simulink model "nav_leha19b"  (R2019b)
settings: Solver=FixedStepDiscrete  StartTime=0.0  StopTime=2500  FixedStep=dT  RelTol=1e-3
values from neighbouring files (symbols this model uses):
  al_gp_M = k    (= 2)    [gnss_data_orig.m]
  al_gp_max = 15    [model_nav_system_flight_simulation_orig.m]
  al_gp_mu = 3.986004418E+14    (= 398600441800000)    [gnss_data_orig.m]
  al_gp_resolution = 1000    [gnss_data_orig.m]
  al_gp_t0 = gnss_strings_2(1,4)    [gnss_data_orig.m]
  dT = 1    [model_nav_system_flight_simulation_orig.m]
  mean_p_ion = 1.3    [model_nav_system_flight_simulation_orig.m]
  mean_p_trop = 0.3    [model_nav_system_flight_simulation_orig.m]
  P0_b_g = zeros(23,23)    [model_nav_system_flight_simulation_orig.m]
  P_b = zeros(21, 21)    [model_nav_system_flight_simulation_orig.m]
  R_a = 6378136    [model_nav_system_flight_simulation_orig.m]
  R_betta = 0.0053171    [model_nav_system_flight_simulation_orig.m]
  R_betta1 = 71 * 10^-7    (= 7.1e-06)    [model_nav_system_flight_simulation_orig.m]
  R_e2 = 0    [model_nav_system_flight_simulation_orig.m]
  R_ge = 9.78049    [model_nav_system_flight_simulation_orig.m]
  R_q = 0.00346775    [model_nav_system_flight_simulation_orig.m]
  R_u = 7.292115*10^(-5)    (= 7.292115e-05)    [model_nav_system_flight_simulation_orig.m]
  sigma_error_acs0 = [SKO_del_n_x SKO_del_n_y SKO_del_n_z]    [model_nav_system_flight_simulation_orig.m]
  sigma_error_DUS0 = [SKO_del_Omega_x SKO_del_Omega_y SKO_del_Omega_z]    [model_nav_system_flight_simulation_orig.m]
  sigma_gnss0 = SKO_p_del_T + SKO_p_del_t + mean_p_ion + mean_p_trop + SKO_p_mnogoluch + SKO_p_noise    (= 5.61)    [model_nav_system_flight_simulation_orig.m]
  SKO_p_del_T = 3    [model_nav_system_flight_simulation_orig.m]
  SKO_p_del_t = 0.01    [model_nav_system_flight_simulation_orig.m]
  SKO_p_mnogoluch = 0.5    [model_nav_system_flight_simulation_orig.m]
  SKO_p_noise = 0.5    [model_nav_system_flight_simulation_orig.m]
  tr_H = flight_mission(3,1)    [model_nav_system_flight_simulation_orig.m]
  W = W'    [model_nav_system_flight_simulation_orig.m]
  X0 = X0'    [model_nav_system_flight_simulation_orig.m]
  X0_b_g = X0_b_g * 0    [model_nav_system_flight_simulation_orig.m]
undefined symbols (not defined in the file or in its folder): al_gp_e, al_gp_health, al_gp_i, al_gp_lan, al_gp_m0, al_gp_sqrt_a, al_gp_w, sigma_error_D_p, sigma_error_D_p1, sigma_gnss0_0, tr_course, tr_fi, tr_la, tr_pitch, tr_roll, tr_V_E, tr_V_H, tr_V_N, tr_X_dgsk, tr_Y_dgsk, tr_Z_dgsk
libraries: simulink_extras x8
(part 2 of 3)

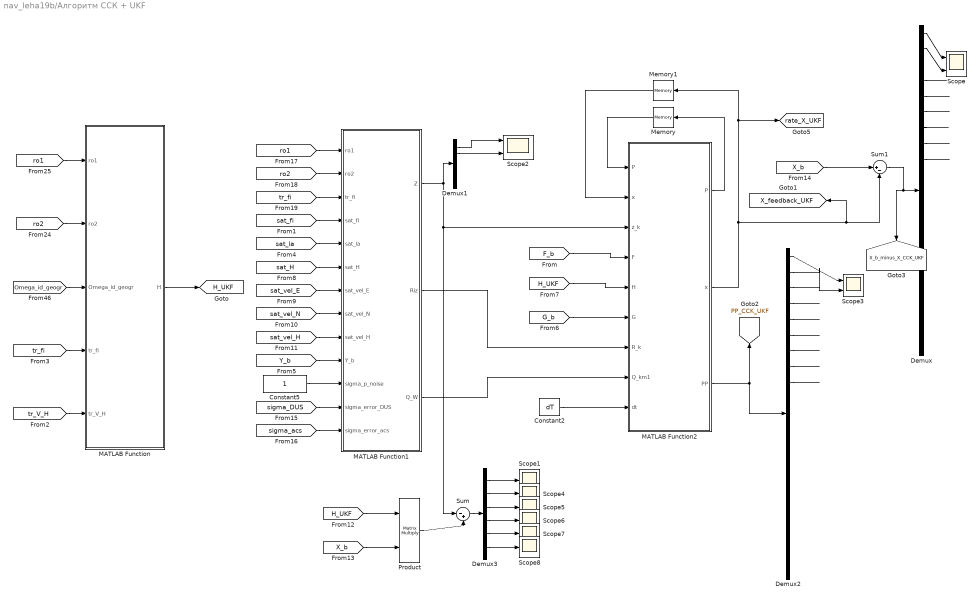
== system nav_leha19b/Алгоритм ССК + UKF ==
  Constant2 : Constant  Value=dT
  Constant5 : Constant
  Demux : Demux  Outputs=21
  Demux1 : Demux  Outputs=6
  Demux2 : Demux  Outputs=21
  Demux3 : Demux  Outputs=6
  MATLAB Function : MATLAB Function  TreatAsAtomicUnit=on
  MATLAB Function1 : MATLAB Function  TreatAsAtomicUnit=on
  MATLAB Function2 : MATLAB Function  TreatAsAtomicUnit=on
  Memory : Memory  InitialCondition=P_b
  Memory1 : Memory  InitialCondition=X0
  Product : Product  Multiplication=Matrix(*)
  Scope : Scope  NumInputPorts=2
  Scope{1,4..8} (6 alike) : Scope
  Scope2 : Scope  NumInputPorts=2
  Scope3 : Scope  NumInputPorts=2
  Sum : Sum  Inputs=|-+
  Sum1 : Sum  Inputs=|+-
  tag scope: H_UKF=global, PP_CCK_UKF=global, X_b_minus_X_CCK_UKF=global, X_feedback_UKF=global, rate_X_UKF=global
  wires:
  Constant2/1 -> MATLAB Function2/9(dt)
  [G_b] -> MATLAB Function2/6(G)
  [H_UKF] -> MATLAB Function2/5(H)
  MATLAB Function/1(H) -> [H_UKF]
  [ro2] -> MATLAB Function/2(ro2)
  [ro1] -> MATLAB Function/1(ro1)
  [Omega_id_geogr] -> MATLAB Function/3(Omega_id_geogr)
  [tr_fi] -> MATLAB Function/4(tr_fi)
  [tr_V_H] -> MATLAB Function/5(tr_V_H)
  [Y_b] -> MATLAB Function1/10(Y_b)
  [sigma_DUS] -> MATLAB Function1/12(sigma_error_DUS)
  [sigma_acs] -> MATLAB Function1/13(sigma_error_acs)
  MATLAB Function1/1(Z) -> Demux1/1, Sum/1, MATLAB Function2/3(z_k)
  MATLAB Function1/2(Riz) -> MATLAB Function2/7(R_k)
  MATLAB Function1/3(Q_W) -> MATLAB Function2/8(Q_km1)
  [X_b] -> Sum1/1
  Sum1/1 -> Demux/1, [X_b_minus_X_CCK_UKF]
  [sat_fi] -> MATLAB Function1/4(sat_fi)
  [sat_la] -> MATLAB Function1/5(sat_la)
  [sat_H] -> MATLAB Function1/6(sat_H)
  [sat_vel_N] -> MATLAB Function1/8(sat_vel_N)
  [sat_vel_H] -> MATLAB Function1/9(sat_vel_H)
  [sat_vel_E] -> MATLAB Function1/7(sat_vel_E)
  Constant5/1 -> MATLAB Function1/11(sigma_p_noise)
  Demux1/1 -> Scope2/1
  Demux1/2 -> Scope2/2
  Demux/4 -> ?
  Demux/5 -> ?
  Demux/6 -> ?
  Demux/7 -> ?
  Demux/8 -> ?
  Demux/9 -> ?
  Demux2/1 -> Scope3/1
  Demux2/2 -> Scope3/2
  Demux2/3 -> ?
  Demux2/4 -> ?
  Demux2/5 -> ?
  Demux2/6 -> ?
  Demux2/7 -> ?
  Demux2/8 -> ?
  Demux2/9 -> ?
  Demux/1 -> Scope/1
  Demux/2 -> Scope/2
  Product/1 -> Sum/2
  [H_UKF] -> Product/1
  [X_b] -> Product/2
  Sum/1 -> Demux3/1
  Demux3/1 -> Scope1/1
  Demux3/2 -> Scope4/1
  Demux3/3 -> Scope5/1
  Demux3/4 -> Scope6/1
  Demux3/5 -> Scope7/1
  Demux3/6 -> Scope8/1
  [ro1] -> MATLAB Function1/1(ro1)
  [ro2] -> MATLAB Function1/2(ro2)
  [F_b] -> MATLAB Function2/4(F)
  MATLAB Function2/1(P) -> Memory/1
  Memory/1 -> MATLAB Function2/1("P ")
  MATLAB Function2/2(x) -> [X_feedback_UKF], Sum1/2, Memory1/1, [rate_X_UKF]
  Memory1/1 -> MATLAB Function2/2("x ")
  MATLAB Function2/3(PP) -> Demux2/1, [PP_CCK_UKF]
  [tr_fi] -> MATLAB Function1/3(tr_fi)

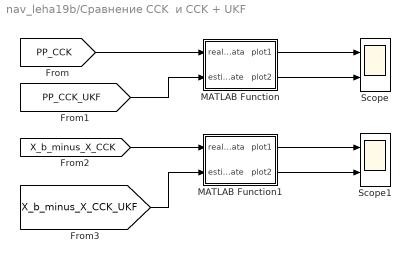
== system nav_leha19b/Сравнение ССK  и CCK + UKF ==
  MATLAB Function : MATLAB Function  TreatAsAtomicUnit=on
  MATLAB Function1 : MATLAB Function  TreatAsAtomicUnit=on
  Scope : Scope  NumInputPorts=2
  Scope1 : Scope  NumInputPorts=2
  wires:
  [PP_CCK] -> MATLAB Function/1(real_data)
  MATLAB Function/1(plot1) -> Scope/1
  [X_b_minus_X_CCK_UKF] -> MATLAB Function1/2(estimate)
  [PP_CCK_UKF] -> MATLAB Function/2(estimate)
  [X_b_minus_X_CCK] -> MATLAB Function1/1(real_data)
  MATLAB Function/2(plot2) -> Scope/2
  MATLAB Function1/1(plot1) -> Scope1/1
  MATLAB Function1/2(plot2) -> Scope1/2

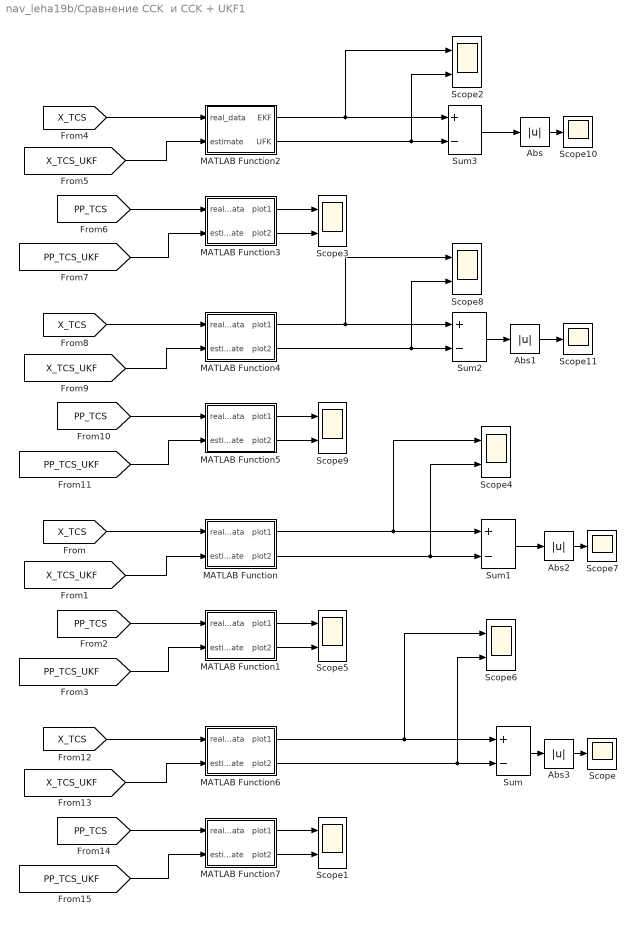
== system nav_leha19b/Сравнение ССK  и CCK + UKF1 ==
  Abs{,1..3} (4 alike) : Abs
  MATLAB Function : MATLAB Function  TreatAsAtomicUnit=on
  MATLAB Function1 : MATLAB Function  TreatAsAtomicUnit=on
  MATLAB Function2 : MATLAB Function  TreatAsAtomicUnit=on
  MATLAB Function3 : MATLAB Function  TreatAsAtomicUnit=on
  MATLAB Function4 : MATLAB Function  TreatAsAtomicUnit=on
  MATLAB Function5 : MATLAB Function  TreatAsAtomicUnit=on
  MATLAB Function6 : MATLAB Function  TreatAsAtomicUnit=on
  MATLAB Function7 : MATLAB Function  TreatAsAtomicUnit=on
  Scope{,7,10..11} (4 alike) : Scope
  Scope{1..6,8..9} (8 alike) : Scope  NumInputPorts=2
  Sum{,1..3} (4 alike) : Sum  Inputs=+-
  wires:
  [PP_TCS] -> MATLAB Function1/1(real_data)
  MATLAB Function1/1(plot1) -> Scope5/1
  MATLAB Function1/2(plot2) -> Scope5/2
  [PP_TCS_UKF] -> MATLAB Function1/2(estimate)
  [X_TCS] -> MATLAB Function/1(real_data)
  [X_TCS_UKF] -> MATLAB Function/2(estimate)
  [X_TCS_UKF] -> MATLAB Function2/2(estimate)
  [PP_TCS_UKF] -> MATLAB Function3/2(estimate)
  [X_TCS] -> MATLAB Function2/1(real_data)
  [PP_TCS] -> MATLAB Function3/1(real_data)
  [X_TCS_UKF] -> MATLAB Function4/2(estimate)
  [PP_TCS_UKF] -> MATLAB Function5/2(estimate)
  [X_TCS] -> MATLAB Function4/1(real_data)
  MATLAB Function5/2(plot2) -> Scope9/2
  MATLAB Function5/1(plot1) -> Scope9/1
  [PP_TCS] -> MATLAB Function5/1(real_data)
  MATLAB Function6/2(plot2) -> Scope6/2, Sum/2
  [X_TCS_UKF] -> MATLAB Function6/2(estimate)
  [PP_TCS_UKF] -> MATLAB Function7/2(estimate)
  [X_TCS] -> MATLAB Function6/1(real_data)
  MATLAB Function6/1(plot1) -> Sum/1, Scope6/1
  [PP_TCS] -> MATLAB Function7/1(real_data)
  MATLAB Function/2(plot2) -> Sum1/2, Scope4/2
  MATLAB Function/1(plot1) -> Sum1/1, Scope4/1
  MATLAB Function4/2(plot2) -> Sum2/2, Scope8/2
  MATLAB Function4/1(plot1) -> Scope8/1, Sum2/1
  MATLAB Function2/2(UFK) -> Sum3/2, Scope2/2
  MATLAB Function2/1(EKF) -> Sum3/1, Scope2/1
  Sum3/1 -> Abs/1
  Abs/1 -> Scope10/1
  Sum2/1 -> Abs1/1
  Abs1/1 -> Scope11/1
  Sum1/1 -> Abs2/1
  Abs2/1 -> Scope7/1
  Abs3/1 -> Scope/1
  Sum/1 -> Abs3/1
  MATLAB Function7/2(plot2) -> Scope1/2
  MATLAB Function7/1(plot1) -> Scope1/1
  MATLAB Function3/2(plot2) -> Scope3/2
  MATLAB Function3/1(plot1) -> Scope3/1

== matlab function nav_leha19b/trajectory/MATLAB Function1 ==
  data: tr_dV_E input; tr_V_E input; tr_dV_N input; tr_V_N input; n_E output; n_N output; tr_dV_H input; n_H output; Omega_E output; Omega_N output; tr_V_H input; tr_fi input; tr_H input; R_ge input; R_betta input; R_betta1 input; R_e2 input; R_a input; R_q input; R_u input; Omega_H output; Omega1_E1 output; Omega1_N1 output; Omega1_H1 output; ro1 output; ro2 output
function [n_E, n_N, n_H, Omega_E, Omega_N, Omega_H, Omega1_E1, Omega1_N1, Omega1_H1, ro1, ro2]  = n(tr_dV_E, tr_V_E, tr_dV_N, tr_V_N, tr_dV_H, tr_V_H, tr_fi, tr_H, R_ge, R_betta, R_betta1, R_e2, R_a, R_q, R_u)

g0 = R_ge*(1 + R_betta*sin(tr_fi).^2 + R_betta1*sin(2*tr_fi).^2);
gy = g0*sin(2*tr_fi)*tr_H*(R_e2/R_a - 2*R_q)/R_a;
gz = g0 + tr_H*(3*tr_H/R_a - 2*R_q*R_ge*cos(tr_fi).^2 + R_e2*(3*sin(tr_fi).^2 - 1) - R_q*(1 + 6*sin(tr_fi).^2))/R_a;

ro1 = (R_a*(1 - R_e2)./(sqrt((1 - R_e2*sin(tr_fi).^2).^3))) + tr_H;
ro2 = (R_a./(sqrt(1 - R_e2*sin(tr_fi).^2))) + tr_H;

Omega1_E = -tr_V_N/ro1;
Omega1_N = tr_V_E/ro2;
Omega1_H = (tr_V_E/ro2)*tan(tr_fi);

u_N = R_u*cos(tr_fi);
u_H = R_u*sin(tr_fi);
Omega_E = Omega1_E;
Omega_N = Omega1_N + u_N;
Omega_H = Omega1_H + u_H;

n_E = tr_dV_E - (Omega1_H + 2*u_H)*tr_V_N + (Omega1_N + 2*u_N)*tr_V_H;
n_N = tr_dV_N + (Omega1_H + 2*u_H)*tr_V_E - Omega1_E*tr_V_H - gy;
n_H = tr_dV_H - (Omega1_N + 2*u_N)*tr_V_E + Omega1_E*tr_V_N - gz;

Omega1_E1 = -(tr_dV_N - tr_V_H*tr_V_N/ro1)/ro1;
Omega1_N1 = (tr_dV_E - R_u*sin(tr_fi)*tr_V_N - tr_V_H*tr_V_E/ro2)/ro2;
Omega1_H1 = (R_u*cos(tr_fi)*tr_V_N + n_E*tan(tr_fi) + tr_V_H*Omega_H +(tr_V_E*tr_V_N)/(ro2*cos(tr_fi).^2))/ro2;
end

== matlab function nav_leha19b/Алгоритм ССК + UKF/MATLAB Function ==
  settings: updateMethod=DISCRETE  sampleTime=dT
  data: ro1 input; H output; ro2 input; Omega_id_geogr input; tr_fi input; tr_V_H input
function H = H_b_gp(ro1, ro2,  Omega_id_geogr,  tr_fi,  tr_V_H)

    H = zeros(6,21);

    H(1,1) = 1 / (ro2 * cos(tr_fi));
    H(2,2) = 1/ro1;
    H(4,1) = - ((tr_V_H/ro2) + Omega_id_geogr(1) * tan(tr_fi));
    H(4,2) = -Omega_id_geogr(3);
    H(4,4) = 1;
    H(5,1) = - tr_V_H/ro1;
    H(5,5) = 1;

end

== matlab function nav_leha19b/trajectory/MATLAB Function2 ==
  data: tr_X_dgsk input; tr_Y_dgsk input; tr_Z_dgsk input; tr_X_dgsk1 output; tr_Y_dgsk1 output; tr_Z_dgsk1 output
function [tr_X_dgsk1, tr_Y_dgsk1, tr_Z_dgsk1] = fcn(tr_X_dgsk, tr_Y_dgsk, tr_Z_dgsk)
persistent i
if isempty (i)
    i = 1;
end
tr_X_dgsk1 = tr_X_dgsk(i);
tr_Y_dgsk1 = tr_Y_dgsk(i);
tr_Z_dgsk1 = tr_Z_dgsk(i);
i = i + 1;
end

== matlab function nav_leha19b/trajectory/MATLAB Function3 ==
  data: tr_fi input; tr_la input; tr_H input; tr_fit output; tr_lat output; tr_Ht output; tr_V_E input; tr_V_Et output; tr_V_N input; tr_V_H input; tr_V_Nt output; tr_V_Ht output; tr_course input; tr_roll input; tr_courset output; tr_yawt output; tr_rollt output; tr_pitch input; tr_pitcht output
function [tr_fit, tr_lat, tr_Ht, tr_V_Et, tr_V_Nt, tr_V_Ht, tr_courset, tr_yawt, tr_rollt, tr_pitcht] = fcn(tr_fi, tr_la, tr_H, tr_V_E, tr_V_N, tr_V_H, tr_course, tr_roll, tr_pitch)
persistent i
if isempty (i)
    i = 1;
end
tr_fit = tr_fi(i);
tr_lat = tr_la(i);
tr_Ht = tr_H(i);
tr_V_Et = tr_V_E(i);
tr_V_Nt = tr_V_N(i);
tr_V_Ht = tr_V_H(i);
tr_courset = tr_course(i);
if tr_course(i) > pi
    tr_yawt = 2*pi - tr_course(i);
else
    tr_yawt = - tr_course(i);
end
tr_rollt = tr_roll(i);
tr_pitcht = tr_pitch(i);

i = i + 1;
end

== matlab function nav_leha19b/trajectory/MATLAB Function4 ==
  settings: updateMethod=DISCRETE
  data: tr_course input; tr_yaw input; n_id_sv output size=[3,1]; tr_roll input; tr_pitch input; n_id_geogr input size=[3,1]; Omega_id_geogr input size=[3,1]; Omega_id_sv output size=[3,1]; C_sv_gor output
function [n_id_sv, Omega_id_sv, C_sv_gor]  = fcn(tr_course, tr_yaw, tr_roll, tr_pitch, n_id_geogr, Omega_id_geogr)
persistent C
if isempty (C)
    C = zeros(3,3);
end
C_sv_gor = zeros(3,3);
%
% C(1,1) = -sin(tr_course)*cos(tr_pitch);
% C(1,2) = sin(tr_course)*sin(tr_pitch)*cos(tr_roll) + cos(tr_course)*sin(tr_roll);
% C(1,3) = -sin(tr_course)*sin(tr_pitch)*sin(tr_roll) + cos(tr_course)*cos(tr_roll);
% C(2,1) = cos(tr_course)*cos(tr_pitch);
% C(2,2) = -cos(tr_course)*sin(tr_pitch)*cos(tr_roll) + sin(tr_course)*sin(tr_roll);
% C(2,3) = cos(tr_course)*sin(tr_pitch)*sin(tr_roll) + sin(tr_course)*cos(tr_roll);
% C(3,1) = sin(tr_pitch);
% C(3,2) = cos(tr_pitch)*cos(tr_roll);
% C(3,3) = -cos(tr_pitch)*sin(tr_roll);
%
C(1,1) = sin(tr_course)*cos(tr_pitch);
C(1,2) = -sin(tr_course)*sin(tr_pitch)*cos(tr_roll) + cos(tr_course)*sin(tr_roll);
C(1,3) = sin(tr_course)*sin(tr_pitch)*sin(tr_roll) + cos(tr_course)*cos(tr_roll);
C(2,1) = cos(tr_course)*cos(tr_pitch);
C(2,2) = -cos(tr_course)*sin(tr_pitch)*cos(tr_roll) - sin(tr_course)*sin(tr_roll);
C(2,3) = cos(tr_course)*sin(tr_pitch)*sin(tr_roll) - sin(tr_course)*cos(tr_roll);
C(3,1) = sin(tr_pitch);
C(3,2) = cos(tr_pitch)*cos(tr_roll);
C(3,3) = -cos(tr_pitch)*sin(tr_roll);
%
C_sv_gor(1,1) = cos(tr_yaw) * cos(tr_pitch);
C_sv_gor(2,1) = sin(tr_pitch);
C_sv_gor(3,1) = - cos(tr_pitch) * sin(tr_yaw);

C_sv_gor(1,2) = - sin(tr_pitch) * cos(tr_yaw) * cos(tr_roll) + sin(tr_yaw) * sin(tr_roll);
C_sv_gor(2,2) = cos(tr_pitch) * cos(tr_roll);
C_sv_gor(3,2) = cos(tr_yaw) * sin(tr_roll) + sin(tr_pitch) * sin(tr_yaw) * cos(tr_roll);

C_sv_gor(1,3) = sin(tr_pitch) * cos(tr_yaw) * sin(tr_roll) + sin(tr_yaw) * cos(tr_roll);
C_sv_gor(2,3) = - cos(tr_pitch) * sin(tr_roll);
C_sv_gor(3,3) = cos(tr_yaw) * cos(tr_roll) - sin(tr_pitch) * sin(tr_yaw) * sin(tr_roll);
%

n_id_sv = (C') * n_id_geogr;
Omega_id_sv = (C') * Omega_id_geogr;
% C_sv_gor = C;
end

== matlab function nav_leha19b/pseudorange/MATLAB Function2 ==
  data: sat_X_dgsk_past input; sat_Y_dgsk_past input; sat_Z_dgsk_past input; D input size=[1,31]; D1 input; see_flag input size=[1,31]; pos_x_dgsk input size=[1,31]; pos_y_dgsk input size=[1,31]; pos_z_dgsk input size=[1,31]; sat_X_dgsk output size=1; vel_Vx_dgsk input; vel_Vy_dgsk input; vel_Vz_dgsk input; LSM_error input; sat_Y_dgsk output size=1; sat_Z_dgsk output size=1; sat_vel_x_dgsk output; sat_vel_y_dgsk output; sat_vel_z_dgsk output; eval_p_del_T output; eval_p_del_T_past input
function [sat_X_dgsk, sat_Y_dgsk, sat_Z_dgsk, sat_vel_x_dgsk, sat_vel_y_dgsk, sat_vel_z_dgsk, eval_p_del_T] = fcn(sat_X_dgsk_past, sat_Y_dgsk_past, sat_Z_dgsk_past, D, D1, see_flag, pos_x_dgsk, pos_y_dgsk, pos_z_dgsk, vel_Vx_dgsk, vel_Vy_dgsk, vel_Vz_dgsk, LSM_error, eval_p_del_T_past)
    persistent i j sat_R_rsu1 sat_R_rsu_k
    sat_N = sum(see_flag);
    sat_H = zeros(sat_N,4);
    sat_Z_pos_er = zeros(sat_N,1);
    sat_Z_vel_er = zeros(sat_N,1);
    D_cal = zeros(sat_N,1);
    D1_cal = zeros(sat_N,1);
    eval_p_del_T = eval_p_del_T_past;
    sat_R_rsu1 = [sat_X_dgsk_past; sat_Y_dgsk_past; sat_Z_dgsk_past];
    sat_R_rsu_k = [10; 10; 10];
    while abs(sat_R_rsu_k(1) - sat_R_rsu1(1)) > LSM_error && abs(sat_R_rsu_k(2) - sat_R_rsu1(2)) > LSM_error && abs(sat_R_rsu_k(3) - sat_R_rsu1(3)) > LSM_error
        i = int8(0);
        j = int8(1);
        sat_R_rsu1 = sat_R_rsu_k;
        while i <= 30
            i = i + 1;
            if see_flag(i) > 0.5
                D_cal(j) = sqrt((pos_x_dgsk(i) - sat_R_rsu1(1))^2 + (pos_y_dgsk(i) - sat_R_rsu1(2))^2 + (pos_z_dgsk(i) - sat_R_rsu1(3))^2);
                sat_Z_pos_er(j) = D(i) - D_cal(j);
                sat_H(j,1) = (pos_x_dgsk(i) - sat_R_rsu1(1))/D_cal(j);
                sat_H(j,2) = (pos_y_dgsk(i) - sat_R_rsu1(2))/D_cal(j);
                sat_H(j,3) = (pos_z_dgsk(i) - sat_R_rsu1(3))/D_cal(j);
                sat_H(j,4) = 1;
                j = j + 1;
            end
        end
        sat_X = inv(sat_H' * sat_H) * sat_H' * sat_Z_pos_er;
        sat_R_rsu_k(1) = sat_R_rsu1(1) - sat_X(1);
        sat_R_rsu_k(2) = sat_R_rsu1(2) - sat_X(2);
        sat_R_rsu_k(3) = sat_R_rsu1(3) - sat_X(3);
        eval_p_del_T = sat_X(4);
    end
    sat_X_dgsk = sat_R_rsu_k(1);
    sat_Y_dgsk = sat_R_rsu_k(2);
    sat_Z_dgsk = sat_R_rsu_k(3);
    %вычисление проекций скорости
    i = int8(0);
    j = int8(1);
    while i <= 30
        i = i + 1;
        if see_flag(i) > 0.5
            D1_cal(j) = ( ( [pos_x_dgsk(i), pos_y_dgsk(i), pos_z_dgsk(i)] - ...
                        [sat_X_dgsk, sat_Y_dgsk, sat_Z_dgsk] ) ./ D(i) ) * [vel_Vx_dgsk(i); vel_Vy_dgsk(i); vel_Vz_dgsk(i)];
            sat_Z_vel_er(j) = D1(i) - D1_cal(j);
            sat_H(j,1) = (- pos_x_dgsk(i) + sat_X_dgsk)/D_cal(j);
            sat_H(j,2) = (- pos_y_dgsk(i) + sat_Y_dgsk)/D_cal(j);
            sat_H(j,3) = (- pos_z_dgsk(i) + sat_Z_dgsk)/D_cal(j);
            sat_H(j,4) = 1;
            j = j + 1;
        end
    end
    sat_X = inv(sat_H' * sat_H) * sat_H' * sat_Z_vel_er;
    sat_vel_x_dgsk = sat_X(1);
    sat_vel_y_dgsk = sat_X(2);
    sat_vel_z_dgsk = sat_X(3);
end

== matlab function nav_leha19b/agp/Перевод из ИСК в ДГСК ==
  data: pos_x_dgsk output; t input; M input; pos_x input; pos_y input; pos_z input; R_u input; pos_y_dgsk output; pos_z_dgsk output
function [pos_x_dgsk, pos_y_dgsk, pos_z_dgsk]  = ISK_to_DGSK(t, M, pos_x, pos_y, pos_z, R_u)
    persistent m A
    
    A = inv([cos(R_u * t), -sin(R_u * t), 0;
            sin(R_u * t), cos(R_u * t), 0;
            0, 0, 1]);
        
    pos_x_dgsk = zeros(1,31);
    pos_y_dgsk = zeros(1,31);
    pos_z_dgsk = zeros(1,31);
    
   % vel_x_dgsk = zeros(1,31);
   % vel_y_dgsk = zeros(1,31);
   % vel_z_dgsk = zeros(1,31);
    m = 1;
    for m = 1:31
        pos_x_dgsk(m) = A(1,1) * pos_x(m) + A(1,2) * pos_y(m) + A(1,3) * pos_z(m);
        pos_y_dgsk(m) = A(2,1) * pos_x(m) + A(2,2) * pos_y(m) + A(2,3) * pos_z(m);
        pos_z_dgsk(m) = A(3,1) * pos_x(m) + A(3,2) * pos_y(m) + A(3,3) * pos_z(m);
        
        %vel_x_dgsk(m) = vel_x(m) - R_u;
        %vel_x_dgsk(m) = A(1,1) * vel_x(m) + A(1,2) * vel_y(m) + A(1,3) * vel_z(m);
        %vel_y_dgsk(m) = A(2,1) * vel_x(m) + A(2,2) * vel_y(m) + A(2,3) * vel_z(m);
        %vel_z_dgsk(m) = A(3,1) * vel_x(m) + A(3,2) * vel_y(m) + A(3,3) * vel_z(m);
    end
end

== matlab function nav_leha19b/agp/keppler ==
  data: t input; M input; t0 input; lan input; pos_x output size=[1,31]; pos_y output size=[1,31]; pos_z output size=[1,31]; i input; w input; e input; sqrt_a input; m0 input; mu input; resolution input; health input; vel_x output; vel_y output; vel_z output
function [pos_x, pos_y, pos_z, vel_x, vel_y, vel_z] = keppler(t, M, t0, lan, i, w, e, sqrt_a, m0, mu, resolution, health)
    persistent k a mt et vt rt ot_x ot_y d_ot_x d_ot_y m
    pos_x = zeros(1,31);
    pos_y = zeros(1,31);
    pos_z = zeros(1,31);
    
    vel_x = zeros(1,31);
    vel_y = zeros(1,31);
    vel_z = zeros(1,31);
    if isempty(k)
        k = 1;
        a = zeros(1,31);
        mt = zeros(1,31);
        et = mt;
        vt = zeros(1,31);
        rt = zeros(1,31);
        ot_x = zeros(1,31);
        ot_y = ot_x;
        d_ot_x = zeros(1,31);
        d_ot_y = d_ot_x;
        
    end

    dt_ = (t - t0);

    for m = 1:M - 1
    
        a(m) = sqrt_a(m)*sqrt_a(m);
    
        mt(m) = m0(m) + dt_ .* sqrt(mu ./ a(m).^3);
    
        et(m) = mt(m);

        for j = 0:(resolution - 1)
         
            et(m) = et(m) - (et(m) - e(m).*sin(et(m)) - mt(m)) / (1 - e(m) .* (cos(et(m))));
    
        end
    
        vt(m) = 2 .* atan2(sqrt(1 + e(m))*sin(et(m)./ 2), sqrt(1-e(m)) * cos(et(m) ./ 2));
        rt(m) = a(m) .* (1 - e(m) .* cos(et(m)));
    
        ot_x(m) = rt(m) .* cos(vt(m));
        ot_y(m) = rt(m) .* sin(vt(m));
        
        d_ot_x(m) = (sqrt(mu .* a(m)) ./ rt(m)) .* (-sin(et(m)));
        d_ot_y(m) = (sqrt(mu .* a(m)) ./ rt(m)) .* (sqrt(1 - e(m) .^2 ) * cos(et(m)));
    
        pos = [(ot_x(m).*(cos(w(m)).*cos(lan(m)) - sin(w(m)).*cos(i(m)).*sin(lan(m))) - ot_y(m).*(sin(w(m)).*cos(lan(m)) + cos(w(m)).*cos(i(m)).*sin(lan(m)))); 
                (ot_x(m).*(cos(w(m)).*sin(lan(m)) + sin(w(m)).*cos(i(m)).*cos(lan(m))) + ot_y(m).*(cos(w(m)).*cos(i(m)).*cos(lan(m)) - sin(w(m)).*sin(lan(m)))); 
                (ot_x(m).*(sin(w(m)).*sin(i(m))) + ot_y(m).*(cos(w(m)).*sin(i(m))))];
        
        vel = [(d_ot_x(m).*(cos(w(m)).*cos(lan(m)) - sin(w(m)).*cos(i(m)).*sin(lan(m))) - d_ot_y(m).*(sin(w(m)).*cos(lan(m)) + cos(w(m)).*cos(i(m)).*sin(lan(m)))); 
                (d_ot_x(m).*(cos(w(m)).*sin(lan(m)) + sin(w(m)).*cos(i(m)).*cos(lan(m))) + d_ot_y(m).*(cos(w(m)).*cos(i(m)).*cos(lan(m)) - sin(w(m)).*sin(lan(m)))); 
                (d_ot_x(m).*(sin(w(m)).*sin(i(m))) + d_ot_y(m).*(cos(w(m)).*sin(i(m))))];
            
        vel_x(m) = vel(1,1);
        vel_y(m) = vel(2,1);
        vel_z(m) = vel(3,1);
        
        pos_x(m) = pos(1,1);
        pos_y(m) = pos(2,1);
        pos_z(m) = pos(3,1);
    end
end

== matlab function nav_leha19b/pseudorange/azimut ==
  data: tr_X_dgsk input; El output; tr_Y_dgsk input; tr_Z_dgsk input; pos_x_dgsk input; pos_y_dgsk input; pos_z_dgsk input; az output; del_mask input; see_flag output int8; al_gp_health input int8; m output
function [El, az, see_flag, m] = fcn(tr_X_dgsk, tr_Y_dgsk, tr_Z_dgsk, pos_x_dgsk, pos_y_dgsk, pos_z_dgsk, del_mask, al_gp_health)
    %Парусников МГУ стр. 44
    persistent i
    R_g = sqrt(tr_X_dgsk^2 + tr_Y_dgsk^2);
    R = sqrt(tr_X_dgsk^2 + tr_Y_dgsk^2 + tr_Z_dgsk^2);
    A_see_flag = zeros(3,3);
    A_see_flag(1,1) = - tr_Y_dgsk / R_g;
    A_see_flag(1,2) = tr_X_dgsk / R_g;
    A_see_flag(2,1) = (- tr_X_dgsk * tr_Z_dgsk) / (R_g * R);
    A_see_flag(2,2) = (- tr_Y_dgsk * tr_Z_dgsk) / (R_g * R);
    A_see_flag(2,3) = R_g / R;
    A_see_flag(3,1) = tr_X_dgsk / R_g;
    A_see_flag(3,2) = tr_Y_dgsk / R_g;
    A_see_flag(3,3) = tr_Z_dgsk / R_g;
    El = zeros(1,31);
    az = zeros(1,31);
    see_flag = int8(zeros(1,31));
    for i = 1:1:31
        R_s__r = zeros(3,1);

        R_s__r(1,1) = pos_x_dgsk(1,i) - tr_X_dgsk;
        R_s__r(2,1) = pos_y_dgsk(1,i) - tr_Y_dgsk;
        R_s__r(3,1) = pos_z_dgsk(1,i) - tr_Z_dgsk;
        R_s_r = A_see_flag * R_s__r;
    
        if R_g == 0
            error('Углы неопределены');
        end
        sin_El = R_s_r(3) / sqrt(R_s_r(1)^2 + R_s_r(2)^2 + R_s_r(3)^2);
        cos_El = sqrt(1 - sin_El^2);
        if sin_El == 1
            El(1,i) = pi/2;
        else
            El(1,i) = atan(sin_El / cos_El);
        end
        if R_s_r(2) == 0
            if R_s_r(1) > 0
                az(1,i) = pi/2;
            else
                az(1,i) = 3*pi/2;
            end
        else
            az(1,i) = atan (R_s_r(1) / R_s_r(2));
        end
        if R_s_r(2) < 0
                az(1,i) = az(1,i) + pi;
        else
                az(1,i) = az(1,i) + 2 * pi;
        end
        if  El(1,i) < del_mask || al_gp_health(i) > 0.5
            az(1,i) = NaN;
            El(1,i) = NaN;
            see_flag(i) = int8(0);
        else
            see_flag(i) = int8(1);
        end
    end
    m = sum(see_flag);
end

== matlab function nav_leha19b/pseudorange/pseudorange ==
  data: tr_X_dgsk input; D output size=[1,31]; tr_Y_dgsk input; tr_Z_dgsk input; tr_Vx_dgsk input; tr_Vy_dgsk input; tr_Vz_dgsk input; pos_x_dgsk input; pos_y_dgsk input; pos_z_dgsk input; vel_x_dgsk input; vel_y_dgsk input; vel_z_dgsk input; El input; see_flag input int8; D_p output; D1 output; D1_p output; SKO_p_del_T input; SKO_p_del_t input; mean_p_ion input; mean_p_trop input; SKO_p_mnogoluch input; SKO_p_noise input; del_mask input; del_D_p output
function [D, D_p, D1, D1_p, del_D_p] = pseudorange(tr_X_dgsk, tr_Y_dgsk, tr_Z_dgsk, tr_Vx_dgsk, tr_Vy_dgsk, tr_Vz_dgsk, pos_x_dgsk, pos_y_dgsk, pos_z_dgsk, vel_x_dgsk, vel_y_dgsk, vel_z_dgsk, El, see_flag, SKO_p_del_T, SKO_p_del_t, mean_p_ion, mean_p_trop, SKO_p_mnogoluch, SKO_p_noise, del_mask)
    persistent i
    D = zeros(1,31);
    D_p = zeros(1,31);
    D1 = zeros(1,31);
    D1_p = zeros(1,31);
    del_D_p = zeros(1,31);
    del_D1_p = zeros(1,31);
    p_noise = zeros(1,31);
    p_mnogoluch = zeros(1,31);
    p_trop = zeros(1,31);
    p_ion = zeros(1,31);
    p_del_T = zeros(1,31);
    p_del_t = zeros(1,31);
%     p_del_T = 0; %SKO_p_del_T;
%     p_del_t = 0; %SKO_p_del_t;

    for i = 1:1:31
        if see_flag(i) > 0.5
            %дальность до НКА:
            D(i) = sqrt( ( pos_x_dgsk(i) - tr_X_dgsk)^2 + ( pos_y_dgsk(i) - tr_Y_dgsk)^2 + (pos_z_dgsk(i) - tr_Z_dgsk)^2 );
            %псевдодальность: 
%             p_mnogoluch(i) = 0;%abs(normrnd(0,SKO_p_mnogoluch));
            p_noise(i) = SKO_p_noise*randn();
            p_mnogoluch(i) = SKO_p_mnogoluch*randn();
%             p_del_T(i)= SKO_p_del_T*randn;
%             p_del_t(i) = SKO_p_del_t*randn;
%             p_noise(i) = normrnd(0,SKO_p_noise);
%             p_trop(i) = abs((mean_p_trop * 0.707) / sin(El(i)));
%             p_ion(i) = abs((mean_p_ion * 0.707) / sin(El(i)));
            
            del_D_p(i) = p_mnogoluch(i) + p_noise(i); %+ p_trop(i) + p_ion(i)+ p_del_T(i) ;
            
            D_p(i) = D(i) + del_D_p(i);
            del_D1_p(i) = 0;%p_del_t(i);
            %псевдоскорость
            D1(i) = (((pos_x_dgsk(i) - tr_X_dgsk) .* (vel_x_dgsk(i) - tr_Vx_dgsk)) + ...
                        ( (pos_y_dgsk(i) - tr_Y_dgsk) .* (vel_y_dgsk(i) - tr_Vy_dgsk)) + ...
                        ( (pos_z_dgsk(i) - tr_Z_dgsk) .* (vel_z_dgsk(i) - tr_Vz_dgsk))) ./ D(i);
            D1_p(i) = (((pos_x_dgsk(i) - tr_X_dgsk) .* (vel_x_dgsk(i) - tr_Vx_dgsk)) + ...
                        ( (pos_y_dgsk(i) - tr_Y_dgsk) .* (vel_y_dgsk(i) - tr_Vy_dgsk)) + ...
                        ( (pos_z_dgsk(i) - tr_Z_dgsk) .* (vel_z_dgsk(i) - tr_Vz_dgsk))) ./ D_p(i);
        end
    end

end

== matlab function nav_leha19b/error model INS/MATLAB Function ==
  data: b_yaw output; b_la output; X input; b_fi output; tr_fi input; tr_la input; tr_H input; tr_V_E input; tr_V_N input; tr_V_H input; tr_yaw input; tr_course input; tr_roll input; tr_pitch input; b_H output; b_V_E output; b_V_N output; b_V_H output; b_roll output; b_course output; b_pitch output; ro1 input; ro2 input; Omega_id_geogr input; del_b_la output; del_b_fi output; del_b_H output; del_b_V_E output; del_b_V_N output; del_b_V_H output; b_X_dgsk output; b_Y_dgsk output; b_Z_dgsk output; R_a input; R_e2 input; b_V_1 output; b_V_2 output; b_V_3 output; tr_X_dgsk output; tr_Y_dgsk output; tr_Z_dgsk output; R1 output; del_angles output
function [b_yaw, b_la, b_fi, b_H, b_V_E, b_V_N, b_V_H, b_roll, b_course, b_pitch, del_b_la, del_b_fi, del_b_H, del_b_V_E, del_b_V_N, del_b_V_H, b_X_dgsk, b_Y_dgsk, b_Z_dgsk, b_V_1, b_V_2, b_V_3, tr_X_dgsk, tr_Y_dgsk, tr_Z_dgsk, R1, del_angles] = fcn(X, tr_fi, tr_la, tr_H, tr_V_E, tr_V_N, tr_V_H, tr_yaw, tr_course, tr_roll, tr_pitch, ro1, ro2, Omega_id_geogr, R_a, R_e2)

    del_b_la = X(1) ./ ( ro2 .* cos(tr_fi) );
    del_b_fi = X(2) ./ ro1;
    del_b_H = X(3);
    
    del_b_V_E = X(4) - ( (tr_V_H ./ ro2) + Omega_id_geogr(1) .* tan(tr_fi) ) .* X(1) - Omega_id_geogr(3) .* X(2);
    del_b_V_N = X(5) - ( tr_V_H ./ ro1 ) .* X(1);
    del_b_V_H = X(6);

    alpha_1 = - X(2) ./ ro1;
    betta_1 = X(1) ./ ro2;
    gamma_1 = betta_1 .* tan(tr_fi);
    alpha_2 = (7) + alpha_1;
    betta_2 = X(8) + betta_1;
    gamma_2 = X(9) + gamma_1;
    
%     del_roll = ( - sin(tr_course) ./ cos(tr_pitch)) .* alpha_2 + ( cos(tr_course) ./ cos(tr_pitch)) .* betta_2;
     del_course = ( sin(tr_roll) * cos(tr_course) + cos(tr_roll) * sin(tr_course) * tan(tr_pitch)) * alpha_2 + ...
                ( sin(tr_roll) * sin(tr_course) - cos(tr_roll) * cos(tr_course) * tan(tr_pitch)) * betta_2 + ...
                cos(tr_roll) * gamma_2;
%     del_pitch = ( cos(tr_roll) * cos(tr_course) - sin(tr_roll) * sin(tr_course) * tan(tr_pitch)) * alpha_2 + ...
%                 ( cos(tr_roll) * sin(tr_course) + sin(tr_roll) * cos(tr_course) * tan(tr_pitch)) * betta_2 - ...
%                 sin(tr_roll) * gamma_2;
            
    del_angles = [sin(tr_yaw) * tan(tr_pitch), cos(tr_yaw) * tan(tr_pitch), -1; cos(tr_yaw), - sin(tr_yaw), 0; sin(tr_yaw)/cos(tr_pitch), cos(tr_pitch)/cos(tr_pitch), 0] * ...
                 [alpha_2; betta_2; gamma_2];

    b_yaw = tr_yaw + del_angles(1);
        
    b_la = tr_la + del_b_la;
    b_fi = tr_fi + del_b_fi;
    b_H = tr_H + del_b_H;
    b_V_E = tr_V_E + del_b_V_E;
    b_V_N = tr_V_N + del_b_V_N;
    b_V_H = tr_V_H + del_b_V_H;
    b_roll = tr_roll + del_angles(3);
    b_course = 0; tr_course + del_course;
    b_pitch = tr_pitch + del_angles(2);
    
    R1 = R_a / sqrt(1 - R_e2 * (sin(tr_fi) ^ 2));

    tr_X_dgsk = (tr_H + R1) * cos(tr_fi) * cos(tr_la);
    tr_Y_dgsk = (tr_H + R1) * cos(tr_fi) * sin(tr_la);
    tr_Z_dgsk = ((1 - R_e2) * R1 + tr_H) * sin(tr_fi);
    
    R1 = R_a / sqrt(1 - R_e2 * (sin(tr_fi) ^2 )); 

    b_X_dgsk = (b_H + R1) * cos(b_fi) * cos(b_la);
    b_Y_dgsk = (b_H + R1) * cos(b_fi) * sin(b_la);
    b_Z_dgsk = ((1 - R_e2) * R1 + b_H) * sin(b_fi);
    
    B = [ -sin(tr_la), cos(tr_la), 0;
        -cos(tr_la) * sin(tr_fi), -sin(tr_la) * sin(tr_fi), cos(tr_fi);
        cos(tr_la) * cos(tr_fi), sin(tr_la) * cos(tr_fi), sin(tr_fi)];
    b_V = (B') * [b_V_E; b_V_N; b_V_H];
    
    b_V_1 = b_V(1);
    b_V_2 = b_V(2);
    b_V_3 = b_V(3);
    
    %ro11 = (R_a*(1 - R_e2)./(sqrt((1 - R_e2*sin(b_fi).^2).^3))) + b_H;
    %ro21 = (R_a./(sqrt(1 - R_e2*sin(b_fi).^2))) + b_H;
end

== matlab function nav_leha19b/error model INS/MATLAB Function3 ==
  data: X_past input; dT input; C_sv_gor input size=[3,3]; X output; n_id_geogr input; Omega_id_geogr input; Omega1 input; n_id_sv input; Omega_id_sv input; W input size=[6,1]; F_b output; G_b output
function [X, F_b, G_b] = INS_error_model(X_past, dT, C_sv_gor, n_id_geogr, Omega_id_geogr, Omega1, n_id_sv, Omega_id_sv, W)
persistent w0 F G 
if isempty(w0)
    w0 = 1.25 * 10^-3;  %частота Шулера [1/c]
    F = zeros(21,21);
    G = zeros(21,6);
end


F(1,4) = 1;
F(2,5) = 1;
F(4,1) = -w0^2 + Omega_id_geogr(2).^2 + Omega_id_geogr(3).^2;
F(4,2) = Omega1(3) - Omega_id_geogr(1)*Omega_id_geogr(2);
F(4,3) = -(Omega1(2) + Omega_id_geogr(1)*Omega_id_geogr(3));
F(4,5) = 2*Omega_id_geogr(3);
F(4,6) = -2*Omega_id_geogr(2);
F(4,8) = n_id_geogr(3);
F(4,9) = - n_id_geogr(2);
F(4,16) = C_sv_gor(1,1);
F(4,17) = C_sv_gor(1,2);
F(4,18) = C_sv_gor(1,3);
F(4,19) = n_id_sv(1)*C_sv_gor(1,1);
F(4,20) = n_id_sv(2)*C_sv_gor(1,2);
F(4,21) = n_id_sv(3)*C_sv_gor(1,3);
F(5,1) = -(Omega1(3) - Omega_id_geogr(1)*Omega_id_geogr(2));
F(5,2) = -w0^2 + Omega_id_geogr(1).^2 + Omega_id_geogr(2).^2;
F(5,3) = Omega1(1) - Omega_id_geogr(2)*Omega_id_geogr(3);
F(5,4) = -2*Omega_id_geogr(3);
F(5,5) = 0;
F(5,6) = 2*Omega_id_geogr(1);
F(5,7) = -n_id_geogr(3);
F(5,9) = n_id_geogr(1);
F(5,16) = C_sv_gor(2,1);
F(5,17) = C_sv_gor(2,2);
F(5,18) = C_sv_gor(2,3);
F(5,19) = n_id_sv(1)*C_sv_gor(2,1);
F(5,20) = n_id_sv(2)*C_sv_gor(2,2);
F(5,21) = n_id_sv(3)*C_sv_gor(2,3);
F(7,8) = Omega_id_geogr(3);
F(7,9) = - Omega_id_geogr(2);
F(7,10) = C_sv_gor(1,1);
F(7,11) = C_sv_gor(1,2);
F(7,12) = C_sv_gor(1,3);
F(7,13) = Omega_id_sv(1)*C_sv_gor(1,1);
F(7,14) = Omega_id_sv(2)*C_sv_gor(1,2);
F(7,15) = Omega_id_sv(3)*C_sv_gor(1,3);
F(8,7) = -Omega_id_geogr(3);
F(8,9) = Omega_id_geogr(1);
F(8,10) = C_sv_gor(2,1);
F(8,11) = C_sv_gor(2,2);
F(8,12) = C_sv_gor(2,3);
F(8,13) = Omega_id_sv(1)*C_sv_gor(2,1);
F(8,14) = Omega_id_sv(2)*C_sv_gor(2,2);
F(8,15) = Omega_id_sv(3)*C_sv_gor(2,3);
F(9,7) = Omega_id_geogr(2);
F(9,8) = -Omega_id_geogr(1);
F(9,10) = C_sv_gor(3,1);
F(9,11) = C_sv_gor(3,2);
F(9,12) = C_sv_gor(3,3);
F(9,13) = Omega_id_sv(1)*C_sv_gor(3,1);
F(9,14) = Omega_id_sv(2)*C_sv_gor(3,2);
F(9,15) = Omega_id_sv(3)*C_sv_gor(3,3);

G(4,4) = C_sv_gor(1,1); 
G(4,5) = C_sv_gor(1,2);
G(4,6) = C_sv_gor(1,3);
G(5,4) = C_sv_gor(2,1);
G(5,5) = C_sv_gor(2,2);
G(5,6) = C_sv_gor(2,3);
G(7,1) = C_sv_gor(1,1);
G(7,2) = C_sv_gor(1,2);
G(7,3) = C_sv_gor(1,3);
G(8,1) = C_sv_gor(2,1);
G(8,2) = C_sv_gor(2,2);
G(8,3) = C_sv_gor(2,3);
G(9,1) = C_sv_gor(3,1);
G(9,2) = C_sv_gor(3,2);
G(9,3) = C_sv_gor(3,3);
%%
F_b = F;
G_b = G;
dX = F*X_past + G*W;
X = X_past + dX*dT;
end

== matlab function nav_leha19b/prediction /prediction ==
  data: b_X_dgsk input; b_Y_dgsk input; b_D_p output; b_Z_dgsk input; b_D1_p output; b_V_1 input; b_V_2 input; b_V_3 input; pos_x_dgsk input; pos_y_dgsk input; pos_z_dgsk input; vel_x_dgsk input; vel_y_dgsk input; vel_z_dgsk input; see_flag input
function [b_D_p, b_D1_p] = fcn(b_X_dgsk, b_Y_dgsk, b_Z_dgsk, b_V_1, b_V_2, b_V_3, pos_x_dgsk, pos_y_dgsk, pos_z_dgsk, vel_x_dgsk, vel_y_dgsk, vel_z_dgsk, see_flag)
    persistent i
    b_D_p = zeros(31,1);
    b_D1_p = zeros(31,1);
    for i = 1:1:31
        if see_flag(i) > 0.5
            b_D_p(i) = sqrt ( (pos_x_dgsk(i) - b_X_dgsk).^2 + (pos_y_dgsk(i) - b_Y_dgsk).^2 + (pos_z_dgsk(i) - b_Z_dgsk).^2 );
            b_D1_p(i) = (((pos_x_dgsk(i) - b_X_dgsk) .* (vel_x_dgsk(i) - b_V_1)) + ...
                        ( (pos_y_dgsk(i) - b_Y_dgsk) .* (vel_y_dgsk(i) - b_V_2)) + ...
                        ( (pos_z_dgsk(i) - b_Z_dgsk) .* (vel_z_dgsk(i) - b_V_3))) ./ b_D_p(i);
        else
            b_D_p(i) = NaN;
            b_D1_p(i) = NaN;
        end
    end
end

== matlab function nav_leha19b/prediction /MATLAB Function1 ==
  settings: updateMethod=DISCRETE  sampleTime=dT
  data: b_D_p input; Z_b_g output double size=[2*al_gp_max,1]; b_D1_p input; D_p input; D1_p input; see_flag input; al_gp_max input
function Z_b_g  = fcn(b_D_p, b_D1_p, D_p, D1_p, see_flag, al_gp_max)
    persistent i j m
    m = sum(see_flag);

    Z_b_g = zeros(2 * al_gp_max, 1);

    i = int8(1);
    for j = 1:1:31
        if see_flag(j) == 1
            Z_b_g(i) = b_D_p(j) - D_p(j);
            i = i + 1;
        end
    end
    i = int8(m + 1 + (al_gp_max - m));
    for j = 1:1:31
        if see_flag(j) == 1
            Z_b_g(i) = b_D1_p(j) - D1_p(j);
            i = i + 1;
        end
    end
%     %вырезаем пустные элементы Z_b_g
%     j = 0;
%     k = length(Z_b_g);
%     for ii = 1:1:((al_gp_max - m) * 2)
%         Z_b_g(k - j) = [];
%         j = j + 1;
%     end
    %Z1 = zeros(al_gp_max, 1);
    %Z2 = zeros(al_gp_max, 1);

%     Z1 = Z_b_g(1:al_gp_max);
%     Z2 = Z_b_g(al_gp_max + 1:2 * al_gp_max);
%     Z1 = Z_b_g(1);
%     Z2 = Z_b_g(16);
end

== matlab function nav_leha19b/Алгоритм ЖСК БИНС + ГНСС/MATLAB Function ==
  settings: updateMethod=DISCRETE  sampleTime=dT
  data: tr_la input; tr_fi input; tr_H input; tr_V_H input; R1 input; ro1 input; H_b_g output size=[2 * al_gp_max, 23]; ro2 input; R_a input; R_e2 input; b_D_p input; pos_x_dgks input; pos_y_dgks input; pos_z_dgks input; b_X_dgsk input; b_Y_dgsk input; b_Z_dgsk input; Omega_id_geogr input; see_flag input; al_gp_max input
function H_b_g = H_b_gp(tr_la, tr_fi, tr_H, tr_V_H, R1, ro1, ro2, R_a, R_e2, b_D_p, pos_x_dgks, pos_y_dgks, pos_z_dgks, b_X_dgsk, b_Y_dgsk, b_Z_dgsk, Omega_id_geogr, see_flag, al_gp_max)
    persistent i j m
    m = sum(see_flag);
    b_la = tr_la;
    b_fi = tr_fi;
    b_H = tr_H;
    b_V_H = tr_V_H;

    Omega_E = Omega_id_geogr(1);
    Omega_N = Omega_id_geogr(2);
    Omega_H = Omega_id_geogr(3);

    i = int8(1);
    j = int8(1);
    
    H_b_g = zeros(2 * al_gp_max, 23);

    while j <= 31
        if see_flag(j) > 0.5
            dR1_db_fi = (R_a * R_e2 * cos(b_fi) * sin(b_fi)) / (( 1 - R_e2 * ((sin(b_fi)) ^ 2)) ^ (3/2));
            
            %Rtp = sin(b_fi) * (R1 + b_H) - cos(b_fi) * dR1_db_fi;
            
            dp_dfi = (1 / b_D_p(j)) * ...
                    ((pos_x_dgks(j) - b_X_dgsk) * (- cos(b_la) * cos(b_fi) * dR1_db_fi + (R1 + b_H) * cos(b_la) * sin(b_fi)) + ...
                     (pos_y_dgks(j) - b_Y_dgsk) * (- sin(b_la) * cos(b_fi) * dR1_db_fi + (R1 + b_H) * sin(b_la) * sin(b_fi)) + ...
                     (pos_z_dgks(j) - b_Z_dgsk) * ( - (1 - R_e2) * sin(b_fi) * dR1_db_fi - ((1 - R_e2) * R1 + b_H) * cos(b_fi)));
            
            dp_dH  = (-1 / b_D_p(j)) * (cos(b_fi) * cos(b_la) * (pos_x_dgks(j) - b_X_dgsk) + ...
                     cos(b_fi) * sin(b_la) * (pos_y_dgks(j) - b_Y_dgsk) + ...
                     sin(b_fi) * (pos_z_dgks(j) - b_Z_dgsk));
                 
            H_b_g(i,1) = (1 / b_D_p(j)) * (sin(b_la) * ... 
                         (pos_x_dgks(j) - b_X_dgsk) - cos(b_la) * (pos_y_dgks(j) - b_Y_dgsk));
            H_b_g(i,2) = (1 / ro1) * dp_dfi;
            H_b_g(i,3) = dp_dH;
            H_b_g(i,22) = -1;
            
            i = i + 1;
            j = j + 1;
        else
            j = j + 1;
        end
    end
    i = int8(m + 1 + (al_gp_max - m));
    j = int8(1);
    while j <= 31
        if see_flag(j) > 0.5
            dp1_db_V_E = (1 / b_D_p(j)) * (sin(b_la) * (pos_x_dgks(j) - b_X_dgsk) - ...
            cos(b_la) * (pos_y_dgks(j) - b_Y_dgsk)); %* del_b_V_E;
        
            dp1_db_V_N = (1 / b_D_p(j)) * (cos(b_la) * sin(b_fi) * (pos_x_dgks(j) - b_X_dgsk) + ...
            sin(b_la) * sin(b_fi) * (pos_y_dgks(j) - b_Y_dgsk) - cos(b_fi) * (pos_z_dgks(j) - b_Z_dgsk));% * del_b_V_N;
            
            dp1_db_V_H = (- 1 / b_D_p(j)) * (cos(b_la) * cos(b_fi) * (pos_x_dgks(j) - b_X_dgsk) + ...
            sin(b_la) * cos(b_fi) * (pos_y_dgks(j) - b_Y_dgsk) + sin(b_fi) * (pos_z_dgks(j) - b_Z_dgsk));% * del_b_V_H;
        
            H_b_g(i,1) = - ((b_V_H / ro2) + Omega_E * tan(b_fi)) * dp1_db_V_E;
            H_b_g(i,2) = - Omega_H * dp1_db_V_E - (b_V_H / ro1) * dp1_db_V_N;
            H_b_g(i,3) = Omega_N * dp1_db_V_E - Omega_E * dp1_db_V_N;
            H_b_g(i,4) = dp1_db_V_E;
            H_b_g(i,5) = dp1_db_V_N;
            H_b_g(i,6) = dp1_db_V_H;
            H_b_g(i,23) = 1;
            
            i = i + 1;
            j = j + 1;
        else
            j = j + 1;
        end
    end

end

== matlab function nav_leha19b/Алгоритм ССК/MATLAB Function ==
  settings: updateMethod=DISCRETE  sampleTime=dT
  data: ro1 input; H output; ro2 input; Omega_id_geogr input; tr_fi input; tr_V_H input
function H = H_b_gp(ro1, ro2,  Omega_id_geogr,  tr_fi,  tr_V_H)

    H = zeros(6,21);

    H(1,1) = 1 / (ro2 * cos(tr_fi));
    H(2,2) = 1/ro1;
    H(4,1) = - ((tr_V_H/ro2) + Omega_id_geogr(1) * tan(tr_fi));
    H(4,2) = -Omega_id_geogr(3);
    H(4,4) = 1;
    H(5,1) = - tr_V_H/ro1;
    H(5,5) = 1;

end

== matlab function nav_leha19b/pseudorange/MATLAB Function1 ==
  data: sat_X_dgsk input; sat_fi output; sat_Y_dgsk input; sat_Z_dgsk input; sat_vel_x_dgsk input; sat_vel_y_dgsk input; sat_vel_z_dgsk input; sat_la output; sat_H output; ellipse_mode input; sat_vel_E output; sat_vel_N output; sat_vel_H output
function [sat_fi, sat_la, sat_H, sat_vel_E, sat_vel_N, sat_vel_H] = fcn(sat_X_dgsk, sat_Y_dgsk, sat_Z_dgsk, sat_vel_x_dgsk, sat_vel_y_dgsk, sat_vel_z_dgsk, ellipse_mode)
    if ellipse_mode == 0
        sat_a = 6378136;
        sat_alpha = 0;
    else
        if ellipse_mode == 1
            sat_a = 6378136;
            sat_alpha = 1/298.25784;
        else
            sat_a = 6378137;
            sat_alpha = 1/298.257223563;
        end
    end
    %вычисление происходит согласно справочнику ПЗ-90.11 приложение 1
    sat_e2 = 2 * sat_alpha - sat_alpha ^ 2;
    sat_r = sqrt( sat_X_dgsk ^ 2 + sat_Y_dgsk ^ 2);
    if sat_r == 0
        sat_fi = pi * sat_Z_dgsk / ( 2 * abs(sat_Z_dgsk));
        sat_la = 0;
        sat_H = sat_Z_dgsk * sin(sat_fi) - sat_a * sqrt ( 1 - (sat_e2 ^ 2) * (sin(sat_fi) ^ 2));
    else
        if sat_r > 0
            tr_la_a = abs( asin( sat_Y_dgsk / sat_r));
            if sat_Y_dgsk < 0 && sat_X_dgsk > 0
                sat_la = 2 * pi - tr_la_a;
            else
                if sat_Y_dgsk < 0 && sat_X_dgsk < 0
                    sat_la = pi + tr_la_a;
                else
                    if sat_Y_dgsk > 0 && sat_X_dgsk < 0
                        sat_la = pi - tr_la_a;
                    else
                        sat_la = tr_la_a;
                    end
                end
            end
        else
            sat_la = 999;
        end
    end
    if sat_Z_dgsk == 0
        sat_fi = 0;
        sat_H = sat_r - sat_alpha;
    else
        sat_ro = sqrt ( sat_X_dgsk ^ 2 + sat_Y_dgsk ^ 2 + sat_Z_dgsk ^ 2 );
        sat_c = asin ( sat_Z_dgsk / sat_ro );
        sat_p = sat_e2 * sat_a / ( 2 * sat_ro);
        sat_s1 = 0;
        sat_b = sat_c + sat_s1;
        sat_s2 = asin ( (sat_p * sin ( 2 * sat_b) ) / sqrt( 1 - sat_e2 * (sin(sat_b) ^ 2)));
        sat_d = abs(sat_s1 - sat_s2);
        while sat_d > (1 / (360 / 0.0001))
            sat_s1 = sat_s2;
            sat_b = sat_c + sat_s1;
            sat_s2 = asin ( (sat_p * sin ( 2 * sat_b) ) / sqrt( 1 - sat_e2 * (sin(sat_b) ^ 2)));
            sat_d = abs(sat_s1 - sat_s2);
        end
        sat_fi = sat_b;
        sat_H = sat_r * cos(sat_fi) + sat_Z_dgsk * sin(sat_fi) - sat_a * sqrt( 1 - sat_e2 * (sin(sat_b) ^ 2));
    end
    sat_vel = [-sin(sat_la), -cos(sat_la) * sin(sat_fi), cos(sat_la) * cos(sat_fi); 
              cos(sat_la), -sin(sat_la) * sin(sat_fi),  sin(sat_la) * cos(sat_fi);
              0, cos(sat_fi), sin(sat_fi)]' * [sat_vel_x_dgsk; sat_vel_y_dgsk; sat_vel_z_dgsk];
    sat_vel_E = sat_vel(1);
    sat_vel_N = sat_vel(2);
    sat_vel_H = sat_vel(3);
end

== matlab function nav_leha19b/Алгоритм ЖСК БИНС + ГНСС/MATLAB Function3 ==
  data: F_b input size=[21,21]; G_b input; F_b_g output size=[23,23]; G_b_g output
function [F_b_g, G_b_g]  = fcn(F_b, G_b)

    F_b_g = zeros(23,23);
    F_b_g(1:21, 1:21) = F_b;

    G_b_g = zeros(23,6);
    G_b_g(1:21, 1:6) = G_b;
    
end

== matlab function nav_leha19b/Алгоритм ЖСК БИНС + ГНСС/MATLAB Function4 ==
  settings: updateMethod=DISCRETE  sampleTime=dT
  data: P_past input; rate_X_past input; P output size=[23,23]; rate_X21 output size=21; F_b_g input size=[23,23]; G_b_g input; rate_X output size=23; H_b_g input size=[2 * al_gp_max, 23]; Rv_b_g input size=[2 * al_gp_max, 2 * al_gp_max]; Z_b_g input size=[2 * al_gp_max, 1]; Q_W input; dt input; T input; P_pos output size=2; P_angle output size=3; P_vel output size=2; PP output size=23
function [P,  rate_X21, rate_X, P_pos, P_angle, P_vel, PP] = fcn(P_past, rate_X_past, F_b_g, G_b_g, H_b_g, Rv_b_g, Z_b_g, Q_W, dt, T)
   
    % матрицы F и G в дискретном виде
    F_b_g_disc = eye(23,23) + F_b_g * T; %(((F_b_g * T) ^ 2) / 2);
    %G_b_g_disc = inv(F_b_g) * (F_b_g_disc - eye(23,23)) * G_b_g;
    G_b_g_disc = G_b_g * T;
    
    S = F_b_g_disc * P_past  * (F_b_g_disc') + G_b_g_disc * Q_W * (G_b_g_disc');
    K = S * (H_b_g') * inv(H_b_g * S * (H_b_g') + Rv_b_g);
    P = (eye(23,23) - K * H_b_g) * S;
    %B и U нулевые (допущение)
    rate_X = F_b_g_disc * rate_X_past + K * (Z_b_g - H_b_g * F_b_g_disc * rate_X_past);

    P_pos = zeros(2,1);
    P_vel = zeros(2,1); 
    P_angle = zeros(3,1);

    P_pos(1) =  sqrt(P(1,1));
    P_pos(2) =  sqrt(P(2,2));
    P_vel(1) = sqrt(P(4,4));
    P_vel(2) = sqrt(P(5,5));
    P_angle(1) = sqrt(P(7,7));
    P_angle(2) = sqrt(P(8,8));
    P_angle(3) = sqrt(P(9,9));

    rate_X21 = rate_X(1:21);
    PP = zeros(23,1);
    for ii = 1:1:23
        PP(ii) = sqrt(P(ii,ii));
    end
end

== matlab function nav_leha19b/Алгоритм ССК + UKF/MATLAB Function1 ==
  data: ro1 input; ro2 input; tr_fi input; sat_fi input; sat_la input; Z output double size=[6,1]; sat_H input; sat_vel_E input; sat_vel_N input; sat_vel_H input; Y_b input; sigma_p_noise input; sigma_error_DUS input; sigma_error_acs input; Riz output double size=[6,6]; Q_W output double size=[6,6]
function [Z, Riz, Q_W]  = fcn(ro1, ro2, tr_fi, sat_fi, sat_la, sat_H, sat_vel_E, sat_vel_N, sat_vel_H, Y_b, sigma_p_noise, sigma_error_DUS, sigma_error_acs)

b_la = Y_b(1);
b_fi = Y_b(2);
b_H = Y_b(3);
b_V_E = Y_b(4);
b_V_N = Y_b(5);
b_V_H = Y_b(6);

Z = [b_la - sat_la; b_fi - sat_fi; b_H - sat_H; b_V_E - sat_vel_E; b_V_N - sat_vel_N; b_V_H - sat_vel_H];

Riz=zeros(6,6); %матрица интенсивности шумов измерений
Riz(1,1) = (sigma_p_noise / ro1) .^ 2;
Riz(2,2) = (sigma_p_noise / (ro2 * cos(tr_fi))) .^ 2;
Riz(3,3) = sigma_p_noise .^ 2;
Riz(4,4) = sigma_p_noise .^ 2;
Riz(5,5) = sigma_p_noise .^ 2;
Riz(6,6) = sigma_p_noise .^ 2;
Q_W = zeros(6,6);
    for i = 1:1:3
        Q_W(i,i) = sigma_error_DUS(i) .^ 2;
        Q_W(i + 3,i + 3) = sigma_error_acs(i) .^ 2;
    end
end

== matlab function nav_leha19b/Алгоритм ЖСК БИНС + ГНСС/MATLAB Function5 ==
  settings: updateMethod=DISCRETE  sampleTime=dT
  data: sigma_error_D_p input; Rv_b_g output size=[2 * al_gp_max, 2 * al_gp_max]; sigma_error_D_p1 input; sigma_error_DUS input; sigma_error_acs input; SKO_gnss0 input; SKO_gnss0_0 input; sigma_error_DUS0 input; sigma_error_acs0 input; dt input; Q_W output; T input; see_flag input; al_gp_max input
function [Rv_b_g, Q_W]  = fcn(sigma_error_D_p, sigma_error_D_p1, sigma_error_DUS, sigma_error_acs, SKO_gnss0, SKO_gnss0_0, sigma_error_DUS0, sigma_error_acs0, dt, T, see_flag, al_gp_max)
    persistent i j flag0 m
    m = sum(see_flag);
    if isempty(flag0)
        Rv_b_g = zeros(2 * al_gp_max, 2 * al_gp_max);
        Rv_b_g = eye(2 * al_gp_max, 2 * al_gp_max) * 0.01 + Rv_b_g;
        for i = 1:1:m
            Rv_b_g(i,i) = (SKO_gnss0_0 .^ 2)/dt;
        end
        for i = (al_gp_max + 1):1:(2 * m + (al_gp_max - m))
            Rv_b_g(i, i) = (SKO_gnss0_0 .^ 2)/dt;
        end
        Q_W = zeros(6,6);
        for i = 1:1:3
            Q_W(i,i) = (sigma_error_DUS(i) .^ 2)/dt;
            Q_W(i + 3,i + 3) = (sigma_error_acs(i) .^ 2)/dt;
        end
        flag0 = int8(0);
    else
        Rv_b_g = zeros(2 * al_gp_max, 2 * al_gp_max);
        Rv_b_g = eye(2 * al_gp_max, 2 * al_gp_max) * 0.01 + Rv_b_g;
        i = 1;
        for j = 1:1:31
            if see_flag(j) == 1
                Rv_b_g(i,i) = (SKO_gnss0_0 .^ 2)/dt;
                Rv_b_g(m + i + (al_gp_max - m), m + i + (al_gp_max - m)) = (SKO_gnss0_0 .^ 2)/dt;
                i = i + 1;
            end 
        end
        Q_W = zeros(6,6);
        for i = 1:1:3
            Q_W(i,i) = (sigma_error_DUS(i) .^ 2)/dt;
            Q_W(i + 3,i + 3) = (sigma_error_acs(i) .^ 2)/dt;
        end
    end
%     j = 0;
%      for ii = 1:1:((al_gp_max - m) * 2)
%         k = size(Rv_b_g, 1);
%         Rv_b_g(k - j, :) = NaN;
%         %Rv_b_g(24, :) = [];
%         %k = size(Rv_b_g, 2);
%         Rv_b_g(:, k - j) = NaN;
%         j = j + 1;
%     end
end

== matlab function nav_leha19b/Алгоритм ЖСК БИНС + ГНСС/MATLAB Function1 ==
  settings: updateMethod=DISCRETE  sampleTime=dT
  data: H_b_g input size=[2 * al_gp_max, 23]; X input; ZZ output size=[30,1]; al_gp_max input
function ZZ   = fcn(H_b_g, X, al_gp_max)
    XX = zeros(23, 1);
    XX(1:21, 1) = X;
    XX(22,1) = 3;
    XX(23,1) = 0.01;
    ZZ = H_b_g * XX;
    
%     HH = zeros(2, 23);
%     HH(1,:) = H_b_g(1,:);
%     HH(2,:) = H_b_g(16,:);
%     
%     ZZ = HH * XX;
% %     ZZ1 = zeros(al_gp_max, 1);
% %     ZZ2 = zeros(al_gp_max, 1);
% 
% %     ZZ1 = ZZ(1:al_gp_max);
% %     ZZ2 = ZZ(al_gp_max + 1:2 * al_gp_max);
% 
%     ZZ1 = ZZ(1);
%     ZZ2 = ZZ(2);
    end

== matlab function nav_leha19b/Алгоритм ССК/MATLAB Function1 ==
  data: ro1 input; ro2 input; tr_fi input; sat_fi input; sat_la input; Z output double size=[6,1]; sat_H input; sat_vel_E input; sat_vel_N input; sat_vel_H input; Y_b input; sigma_p_noise input; sigma_error_DUS input; sigma_error_acs input; Riz output double size=[6,6]; Q_W output double size=[6,6]
function [Z, Riz, Q_W]  = fcn(ro1, ro2, tr_fi, sat_fi, sat_la, sat_H, sat_vel_E, sat_vel_N, sat_vel_H, Y_b, sigma_p_noise, sigma_error_DUS, sigma_error_acs)

b_la = Y_b(1);
b_fi = Y_b(2);
b_H = Y_b(3);
b_V_E = Y_b(4);
b_V_N = Y_b(5);
b_V_H = Y_b(6);

Z = [b_la - sat_la; b_fi - sat_fi; b_H - sat_H; b_V_E - sat_vel_E; b_V_N - sat_vel_N; b_V_H - sat_vel_H];

Riz=zeros(6,6); %матрица интенсивности шумов измерений
Riz(1,1) = (sigma_p_noise / ro1) .^ 2;
Riz(2,2) = (sigma_p_noise / (ro2 * cos(tr_fi))) .^ 2;
Riz(3,3) = sigma_p_noise .^ 2;
Riz(4,4) = sigma_p_noise .^ 2;
Riz(5,5) = sigma_p_noise .^ 2;
Riz(6,6) = sigma_p_noise .^ 2;
Q_W = zeros(6,6);
    for i = 1:1:3
        Q_W(i,i) = sigma_error_DUS(i) .^ 2;
        Q_W(i + 3,i + 3) = sigma_error_acs(i) .^ 2;
    end
end

== matlab function nav_leha19b/Алгоритм ССК/MATLAB Function4 ==
  settings: updateMethod=DISCRETE  sampleTime=dT
  data: P_past input; rate_X_past input; P output; F_b_g input; G_b_g input; rate_X output; H_b_g input; Rv_b_g input; Z_b_g input; Q_W input; dt input; T input; PP output
function [P, rate_X, PP] = fcn(P_past, rate_X_past, F_b_g, G_b_g, H_b_g, Rv_b_g, Z_b_g, Q_W, dt, T)
   
    % матрицы F и G в дискретном виде
    F_b_g_disc = eye(21,21) + F_b_g * T; %+ (((F_b_g * T) ^ 2) / 2) + (((F_b_g * T) ^ 3) / 6) + ...
                %(((F_b_g * T) ^ 4) / 24) +  + (((F_b_g * T) ^ 5) / 120);
    %G_b_g_disc = inv(F_b_g) * (F_b_g_disc - eye(21,21)) * G_b_g;
    G_b_g_disc = G_b_g * T;
    
    S = F_b_g_disc * P_past  * (F_b_g_disc') + G_b_g_disc * Q_W * (G_b_g_disc');
    K = S * (H_b_g') * inv(H_b_g * S * (H_b_g') + Rv_b_g);
    P = (eye(21,21) - K * H_b_g) * S;
    %B и U нулевые (допущение)
    rate_X = F_b_g_disc * rate_X_past + K * (Z_b_g - H_b_g * F_b_g_disc * rate_X_past);
    PP = zeros(21,1);
    for i = 1:1:21
        PP(i) = sqrt(P(i,i));
    end
end
